simulink model "TV_2021"  (R2017b)
settings: Solver=VariableStepAuto  StartTime=0.0  StopTime=10.0  RelTol=1e-3
undefined symbols (not defined in the file): sigbuilder_block
libraries: simulink x6
(part 4 of 13)

== system TV_2021/If Action Subsystem1/VDC 2018 Complete/Optimization SKF & CKF ==
  RPM_INV1 : Inport
  RPM_INV2 : Inport  Port=2
  Steer_An : Inport  Port=3
  SKF_Initial : Inport  Port=4
  CKF_Initial : Inport  Port=5
  Cte_SKF : Inport  Port=6
  Cte_CKF : Inport  Port=7
  CKF_prev : DataStoreRead  DataStoreName=B
  Constant : Constant  Value=0
  Data Store Memory : DataStoreMemory  ReadBeforeWriteMsg=warning  WriteAfterWriteMsg=warning  WriteAfterReadMsg=warning  ShowAdditionalParam=off
  Data Store Memory1 : DataStoreMemory  DataStoreName=B  ReadBeforeWriteMsg=warning  WriteAfterWriteMsg=warning  WriteAfterReadMsg=warning  ShowAdditionalParam=off
  Data Store Write : DataStoreWrite
  Data Store Write1 : DataStoreWrite  DataStoreName=B
  Derivative : Derivative
  Display : Display
  MATLAB Function : MATLAB Function  TreatAsAtomicUnit=on
  Mux : Mux  Inputs=3
  "SKF_prev " : DataStoreRead
  Saturation : Saturate  UpperLimit=6000  LowerLimit=0
  Scope : Scope
  "Subsystem " : Subsystem
  Switch : Switch  Threshold=900
  SKF_act : Outport
  CKF_act : Outport  Port=2
  wires:
  SKF_Initial/1 -> "Subsystem "/3(SKF_Initial)
  CKF_prev/1 -> "Subsystem "/6("CKF_prev ")
  "Subsystem "/1("SKF_act ") -> SKF_act/1, Data Store Write/1  "SKF"
  Derivative/1 -> Switch/1, Switch/2, Saturation/1, Display/1, "Subsystem "/2(Derivative)  "alpha"
  "SKF_prev "/1 -> "Subsystem "/4(SKF_prev)
  "Subsystem "/2(CKF_act) -> CKF_act/1, Data Store Write1/1  "CKF"
  Cte_CKF/1 -> "Subsystem "/8(Cte_CKF)
  Steer_An/1 -> "Subsystem "/1(Steer_An)
  CKF_Initial/1 -> "Subsystem "/5("CKF_Initial ")
  RPM_INV1/1 -> Mux/1, MATLAB Function/1(RPM_INV1)
  RPM_INV2/1 -> MATLAB Function/2(RPM_INV2)
  Cte_SKF/1 -> "Subsystem "/7(Cte_SKF)
  MATLAB Function/1(RPM) -> Derivative/1  "w (rpm)"
  Mux/1 -> Scope/1
  Saturation/1 -> Mux/2
  Switch/1 -> Mux/3
  Constant/1 -> Switch/3

== system TV_2021/If Action Subsystem1/VDC 2018 Complete/Sensor_DATA ==
  note: [rad/s]
  note: [ºC]
  note: [m/s2]
  note: [m/s2]
  note: [deg]
  note: [N]
  note: [N]
  note: [N]
  note: [N]
  note: [0-1]
  note: [0-1]
  note: [0 or 1]
  note: [0 - Inf]
  note: [rad/s]
  note: [rad/s]
  Steer_Ang : Inport
  "F_Acc " : Inport  Port=2
  R_Acc : Inport  Port=3
  Yaw Rate : Inport  Port=4
  FR_Susp : Inport  Port=5
  FL_Susp : Inport  Port=6
  RR_Susp : Inport  Port=7
  RL_Susp : Inport  Port=8
  Gas Pedal : Inport  Port=9
  Brake Pedal : Inport  Port=10
  Regenerative Enable : Inport  Port=11
  "Power " : Inport  Port=12
  TemperatureIN : Inport  Port=13
  Temperature Motor : Inport  Port=14
  V_eRR : Inport  Port=15
  "V_eRL " : Inport  Port=16
  Steer_ang : Outport
  F_acc : Outport  Port=2
  R_acc : Outport  Port=3
  YawRate : Outport  Port=4
  FR_susp : Outport  Port=5
  FL_susp : Outport  Port=6
  RR_susp : Outport  Port=7
  RL_susp : Outport  Port=8
  Gas_Pedal : Outport  Port=9
  Brake_Pedal : Outport  Port=10
  Reg_Enable : Outport  Port=11
  Power : Outport  Port=12
  TemperatureIGBT : Outport  Port=13
  TemperatureMotor : Outport  Port=14
  "V_eRR " : Outport  Port=15
  V_eRL : Outport  Port=16
  wires:
  RL_Susp/1 -> RL_susp/1
  RR_Susp/1 -> RR_susp/1
  FL_Susp/1 -> FL_susp/1
  FR_Susp/1 -> FR_susp/1
  Steer_Ang/1 -> Steer_ang/1
  R_Acc/1 -> R_acc/1
  "F_Acc "/1 -> F_acc/1
  Gas Pedal/1 -> Gas_Pedal/1
  Brake Pedal/1 -> Brake_Pedal/1
  Regenerative Enable/1 -> Reg_Enable/1
  "Power "/1 -> Power/1
  TemperatureIN/1 -> TemperatureIGBT/1
  "V_eRL "/1 -> V_eRL/1
  V_eRR/1 -> "V_eRR "/1
  Temperature Motor/1 -> TemperatureMotor/1
  Yaw Rate/1 -> YawRate/1

== system TV_2021/If Action Subsystem1/VDC 2018 Complete/Wheel_to_engine ==
  "Fx_FR " : Inport
  "Fx_FL " : Inport  Port=2
  "Fx_RR " : Inport  Port=3
  "Fx_RL " : Inport  Port=4
  Re : Inport  Port=5
  RT : Inport  Port=6
  Add : Sum  Inputs=+-
  Constant : Constant  Value=0
  Constant1 : Constant  Value=0
  Fx_to_engineTqRL : Subsystem
  Fx_to_engineTqRR : Subsystem
  MATLAB Function1 : MATLAB Function  TreatAsAtomicUnit=on
  MATLAB Function2 : MATLAB Function  TreatAsAtomicUnit=on
  Tq_diff : Outport  VectorParamsAs1DForOutWhenUnconnected=on
  Tq_FR : Outport  Port=2
  Tq_FL : Outport  Port=3
  Tq_RR : Outport  Port=4
  Tq_RL : Outport  Port=5
  wires:
  Fx_to_engineTqRR/1(Tq) -> Add/1, Tq_RR/1
  Fx_to_engineTqRL/1(Tq) -> Tq_RL/1, Add/2
  "Fx_FR "/1 -> Tq_FR/1
  "Fx_FL "/1 -> Tq_FL/1
  Re/1 -> Fx_to_engineTqRR/2(Re), Fx_to_engineTqRL/2(Re)
  RT/1 -> Fx_to_engineTqRR/3(RT), Fx_to_engineTqRL/3(RT)
  "Fx_RL "/1 -> MATLAB Function2/2(v)
  "Fx_RR "/1 -> MATLAB Function1/2(v)
  MATLAB Function2/1(value) -> Fx_to_engineTqRL/1(Fx)
  MATLAB Function1/1(value) -> Fx_to_engineTqRR/1(Fx)
  Constant1/1 -> MATLAB Function1/1(cte)
  Constant/1 -> MATLAB Function2/1(cte)
  Add/1 -> Tq_diff/1

== system TV_2021/If Action Subsystem1/VDC 2018 without Longitudinal/Constraints ==
  Tq_FRin : Inport
  Tq_FLin : Inport  Port=2
  Tq_RR_wc : Inport  Port=3
  "Tq_RL_wc " : Inport  Port=4
  "Trans_max_static " : Inport  Port=5
  Trans_max_dynamic : Inport  Port=6
  Power : Inport  Port=7
  Power_limit : Inport  Port=8
  ReductionCte_Power : Inport  Port=9
  ReductionCte_Temperature : Inport  Port=10
  TemperatureIGBT : Inport  Port=11
  TemperatureI_limit_Motor : Inport  Port=12
  TemperatureIMotor : Inport  Port=13
  Temperature_limit_IGBT : Inport  Port=14
  V_eRR : Inport  Port=15
  V_eRL : Inport  Port=16
  Tq_max : Inport  Port=17
  MaxRegTorque : Inport  Port=18
  Bp : Inport  Port=19
  Reg_enable : Inport  Port=20
  Acelerating and braking without Regenerative : Subsystem  TreatAsAtomicUnit=on
  Braking with Regenerative : Subsystem  TreatAsAtomicUnit=on
  Constant : Constant  Value=0
  Constant1 : Constant  Value=0
  If : If  NumInputs=2  IfExpression=u2 == 1 & u1 > 0
  Merge1 : Merge
  Merge2 : Merge
  Tq_FRout : Outport
  "Tq_FLout " : Outport  Port=2
  Tq_RRout : Outport  Port=3
  Tq_RLout : Outport  Port=4
  wires:
  Constant1/1 -> "Tq_FLout "/1
  Constant/1 -> Tq_FRout/1
  Tq_RR_wc/1 -> Braking with Regenerative/2(Tq_RR_wc), Acelerating and braking without Regenerative/16(Tq_RR)
  "Tq_RL_wc "/1 -> Acelerating and braking without Regenerative/17(Tq_RL), Braking with Regenerative/3(Tq_RL_wc)
  Tq_max/1 -> Acelerating and braking without Regenerative/1(Tq_max)
  V_eRL/1 -> Acelerating and braking without Regenerative/3(V_eRL)
  Trans_max_dynamic/1 -> Acelerating and braking without Regenerative/4(Trans_max_dynamic)
  "Trans_max_static "/1 -> Acelerating and braking without Regenerative/5(Trans_max_static)
  Merge2/1 -> Tq_RLout/1
  Merge1/1 -> Tq_RRout/1
  Bp/1 -> If/1
  Reg_enable/1 -> If/2
  V_eRR/1 -> Acelerating and braking without Regenerative/2(V_eRR)
  If/1 -> Braking with Regenerative/Action
  If/2 -> Acelerating and braking without Regenerative/Action
  MaxRegTorque/1 -> Braking with Regenerative/1(MaxRegTorque)
  Tq_FRin/1 -> Acelerating and braking without Regenerative/14(Tq_FR)
  Tq_FLin/1 -> Acelerating and braking without Regenerative/15(Tq_FL)
  ReductionCte_Temperature/1 -> Acelerating and braking without Regenerative/13(ReductionCte_Temperature)
  ReductionCte_Power/1 -> Acelerating and braking without Regenerative/12(ReductionCte_Power)
  TemperatureIGBT/1 -> Acelerating and braking without Regenerative/9(TemperatureIGBT)
  Temperature_limit_IGBT/1 -> Acelerating and braking without Regenerative/8(Temperature_limit_IGBT)
  Power/1 -> Acelerating and braking without Regenerative/7(Power)
  Power_limit/1 -> Acelerating and braking without Regenerative/6(Power_limit)
  Acelerating and braking without Regenerative/2(TQ_RL) -> Merge2/1
  Acelerating and braking without Regenerative/1(TQ_RR) -> Merge1/1
  Braking with Regenerative/1(TQ_RR) -> Merge1/2
  Braking with Regenerative/2(TQ_RL) -> Merge2/2
  TemperatureI_limit_Motor/1 -> Acelerating and braking without Regenerative/10(TemperatureI_limit_Motor)
  TemperatureIMotor/1 -> Acelerating and braking without Regenerative/11(TemperatureMotor)

== system TV_2021/If Action Subsystem1/VDC 2018 without Longitudinal/Driver // CarBehaviours ==
  Tq_FRin : Inport
  Tq_FLin : Inport  Port=2
  Tq_RRin : Inport  Port=3
  "Tq_RLin " : Inport  Port=4
  Bp : Inport  Port=5
  Ap : Inport  Port=6
  Reg_enable : Inport  Port=7
  Ap_Sat_up : Inport  Port=8
  Ap_Sat_down : Inport  Port=9
  Accelerating : Subsystem  TreatAsAtomicUnit=on
  Braking Conditions : If  NumInputs=3  IfExpression=u1>0 & u2==0 & u3==1  ElseIfExpressions=u1>0 & u2==0.02 & u3==0, u1==0.02 & u2==0.02
  Constant : Constant  Value=0
  Constant1 : Constant  Value=0
  Inertia Braking : Subsystem  TreatAsAtomicUnit=on
  Mech_Braking : Subsystem  TreatAsAtomicUnit=on
  Merge : Merge  Inputs=4
  Merge1 : Merge  Inputs=4
  Regenerative+Mech Braking : Subsystem  TreatAsAtomicUnit=on
  Terminator : Terminator
  Terminator1 : Terminator
  Tq_FRout : Outport
  "Tq_FLout " : Outport  Port=2
  Tq_RRout : Outport  Port=3
  Tq_RLout : Outport  Port=4
  out_Throttle : Outport  Port=5
  wires:
  Constant1/1 -> "Tq_FLout "/1
  Constant/1 -> Tq_FRout/1
  Tq_FLin/1 -> Terminator1/1
  Tq_FRin/1 -> Terminator/1
  Merge/1 -> Tq_RRout/1
  Merge1/1 -> Tq_RLout/1
  Bp/1 -> Braking Conditions/1
  Ap/1 -> Accelerating/1(Ap), Braking Conditions/2
  Regenerative+Mech Braking/1("Tq_RR ") -> Merge/1
  Mech_Braking/1("Tq_RR ") -> Merge/2
  Inertia Braking/1("Tq_RR ") -> Merge/3
  Accelerating/1("Tq_RR ") -> Merge/4
  Regenerative+Mech Braking/2(Tq_RL) -> Merge1/1
  Mech_Braking/2(Tq_RL) -> Merge1/2
  Inertia Braking/2(Tq_RL) -> Merge1/3
  Accelerating/2(Tq_RL) -> Merge1/4
  Braking Conditions/1 -> Regenerative+Mech Braking/Action
  Braking Conditions/2 -> Mech_Braking/Action
  Braking Conditions/3 -> Inertia Braking/Action
  Braking Conditions/4 -> Accelerating/Action
  Tq_RRin/1 -> Regenerative+Mech Braking/1(RegTq_RR), Accelerating/4(Tq_RR)
  "Tq_RLin "/1 -> Regenerative+Mech Braking/2(RegTq_RL), Accelerating/5("Tq_RL ")
  Ap_Sat_up/1 -> Accelerating/2("Ap_Sat_up ")
  Ap_Sat_down/1 -> Accelerating/3(Ap_Sat_down)
  Reg_enable/1 -> Braking Conditions/3
  Accelerating/3(Out_Throttle) -> out_Throttle/1

== system TV_2021/If Action Subsystem1/VDC 2018 without Longitudinal/In_Numbers ==
  C-Kamm_Factor : Inport
  Max Regen Torque [Nm] : Inport  Port=2
  Limit Power [kW] : Inport  Port=3
  Limit Temperature IGBT [ºC] : Inport  Port=4
  Limit Temperature Motor [ºC] : Inport  Port=5
  Reduction Power [0-1] : Inport  Port=6
  Reduction Temperature [0-1] : Inport  Port=7
  Steering Saturation (per site) [deg] : Inport  Port=8
  Ap_Sat_Down [-] : Inport  Port=9
  Ap_Sat_Up [-] : Inport  Port=10
  3% difference : Gain  Gain=0.97
  Effective Rolling Radius[inch] : Constant  Value=13
  Engine+Inverter Performance [-] : Constant  Value=0.8
  Maximum Torque per engine [Nm] : Constant  Value=140
  Maximum Transmission Torque Dynamic [Nm] : Constant  Value=140
  Maximum Transmission Torque Static [Nm] : Constant  Value=130
  Transmision Ratio[-] : Constant  Value=4
  inch to m : Gain  Gain=0.0254
  Steer_Sat [deg] : Outport
  Tq_Max [Nm] : Outport  Port=2
  Cornering Kamm_Factor [0-2] : Outport  Port=3
  Transmision_Ratio[-] : Outport  Port=4
  Effective Rolling Radius[m] : Outport  Port=5
  Ap_Sat_down[-] : Outport  Port=6
  Ap_Sat_up[-] : Outport  Port=7
  Engine+Inverter Performance[-] : Outport  Port=8
  Trans_max _static[Nm] : Outport  Port=9
  Trans_max_dynamic [Nm] : Outport  Port=10
  "Power limit [KW] " : Outport  Port=11
  Temperature limit IGBT [ºC] : Outport  Port=12
  Temperature limit Motor [ºC] : Outport  Port=13
  Reduction Power (0-1) : Outport  Port=14
  Reduction Temperature (0-1) : Outport  Port=15
  MaxRegTorque [Nm] : Outport  Port=16
  wires:
  Maximum Torque per engine [Nm]/1 -> Tq_Max [Nm]/1
  Transmision Ratio[-]/1 -> Transmision_Ratio[-]/1
  Effective Rolling Radius[inch]/1 -> inch to m/1
  Maximum Transmission Torque Static [Nm]/1 -> Trans_max _static[Nm]/1
  Maximum Transmission Torque Dynamic [Nm]/1 -> Trans_max_dynamic [Nm]/1
  inch to m/1 -> 3% difference/1
  3% difference/1 -> Effective Rolling Radius[m]/1
  Engine+Inverter Performance [-]/1 -> Engine+Inverter Performance[-]/1
  Max Regen Torque [Nm]/1 -> MaxRegTorque [Nm]/1
  Limit Power [kW]/1 -> "Power limit [KW] "/1
  Limit Temperature IGBT [ºC]/1 -> Temperature limit IGBT [ºC]/1
  Reduction Power [0-1]/1 -> Reduction Power (0-1)/1
  C-Kamm_Factor/1 -> Cornering Kamm_Factor [0-2]/1
  Steering Saturation (per site) [deg]/1 -> Steer_Sat [deg]/1
  Ap_Sat_Up [-]/1 -> Ap_Sat_up[-]/1
  Ap_Sat_Down [-]/1 -> Ap_Sat_down[-]/1
  Reduction Temperature [0-1]/1 -> Reduction Temperature (0-1)/1
  Limit Temperature Motor [ºC]/1 -> Temperature limit Motor [ºC]/1

== system TV_2021/If Action Subsystem1/VDC 2018 without Longitudinal/Kamm Circle Lateral ==
  "N_FR " : Inport
  N_FL : Inport  Port=2
  N_RR : Inport  Port=3
  N_RL : Inport  Port=4
  Fy : Inport  Port=5
  CK_Factor : Inport  Port=6
  Constant : Constant  Value=-1
  Constant1 : Constant  Value=-1
  Kamm_Circle LatD : MATLAB Function  TreatAsAtomicUnit=on
  MATLAB Function1 : MATLAB Function  TreatAsAtomicUnit=on
  MATLAB Function2 : MATLAB Function  TreatAsAtomicUnit=on
  Product : Product
  Product1 : Product
  Fx_FR : Outport
  Fx_FL : Outport  Port=2
  "Fx_RR " : Outport  Port=3
  "Fx_RL " : Outport  Port=4
  wires:
  N_FL/1 -> Fx_FL/1
  "N_FR "/1 -> Fx_FR/1
  N_RL/1 -> Kamm_Circle LatD/2(Fz_L)
  Fy/1 -> Kamm_Circle LatD/3(Fy)
  N_RR/1 -> Kamm_Circle LatD/1(Fz_R)
  Kamm_Circle LatD/1(Fx_R) -> Product/1
  Kamm_Circle LatD/2(Fx_L) -> Product1/1
  CK_Factor/1 -> Product/2, Product1/2
  Product1/1 -> MATLAB Function1/2(v)
  Product/1 -> MATLAB Function2/2(v)
  Constant1/1 -> MATLAB Function2/1(cte)
  MATLAB Function2/1(value) -> "Fx_RR "/1
  Constant/1 -> MATLAB Function1/1(cte)
  MATLAB Function1/1(value) -> "Fx_RL "/1

== system TV_2021/If Action Subsystem1/VDC 2018 without Longitudinal/Lateral Dynamics ==
  F_acc : Inport
  R_acc : Inport  Port=2
  FR_susp : Inport  Port=3
  FL_susp : Inport  Port=4
  RR_susp : Inport  Port=5
  RL_susp : Inport  Port=6
  Gas_pedal : Inport  Port=7
  Brake_pedal : Inport  Port=8
  Constant1 : Constant  Value=0
  Constant2 : Constant  Value=0
  Demux : Demux  Outputs=3
  Demux1 : Demux  Outputs=3
  Fy per wheel : Gain  Gain=1/2
  Gravity : Gain  Gain=1/9.81
  Gravity1 : Gain  Gain=1/9.81
  Product : Product
  Sum : Sum  Inputs=++++
  Sum1 : Sum
  Sum2 : Sum  Inputs=+-
  Terminator{1..6} (6 alike) : Terminator
  N_FR : Outport
  "N_FL " : Outport  Port=2
  "N_RR " : Outport  Port=3
  N_RL : Outport  Port=4
  Fy_R : Outport  Port=5
  Mass [kg] (0,inf) : Outport  Port=6
  Handling [-] (-inf,inf) : Outport  Port=7
  wires:
  Constant2/1 -> "N_FL "/1
  Constant1/1 -> N_FR/1
  FL_susp/1 -> Sum/2
  F_acc/1 -> Demux1/1
  RR_susp/1 -> Sum/3, Sum1/1, "N_RR "/1
  RL_susp/1 -> Sum/4, Sum1/2, N_RL/1
  Gas_pedal/1 -> Terminator4/1
  Brake_pedal/1 -> Terminator5/1
  R_acc/1 -> Demux/1
  Demux/2 -> Sum2/2, Product/1
  Demux/1 -> Terminator6/1
  Demux/3 -> Terminator3/1
  Product/1 -> Fy per wheel/1  "Fy per axe"
  Fy per wheel/1 -> Fy_R/1
  Gravity1/1 -> Product/2
  Sum/1 -> Gravity/1
  FR_susp/1 -> Sum/1
  Sum1/1 -> Gravity1/1
  Gravity/1 -> Mass [kg] (0,inf)/1  "Mass [kg]"
  Demux1/1 -> Terminator1/1
  Demux1/3 -> Terminator2/1
  Demux1/2 -> Sum2/1
  Sum2/1 -> Handling [-] (-inf,inf)/1

== system TV_2021/If Action Subsystem1/VDC 2018 without Longitudinal/Optimization SKF & CKF ==
  RPM_INV1 : Inport
  RPM_INV2 : Inport  Port=2
  CKF_Initial : Inport  Port=3
  Cte_CKF : Inport  Port=4
  CKF_prev : DataStoreRead  DataStoreName=B
  Data Store Memory1 : DataStoreMemory  DataStoreName=B  ReadBeforeWriteMsg=warning  WriteAfterWriteMsg=warning  WriteAfterReadMsg=warning  ShowAdditionalParam=off
  Data Store Write1 : DataStoreWrite  DataStoreName=B
  Derivative : Derivative
  MATLAB Function : MATLAB Function  TreatAsAtomicUnit=on
  "Subsystem " : Subsystem
  CKF_act : Outport
  wires:
  CKF_prev/1 -> "Subsystem "/3("CKF_prev ")
  Derivative/1 -> "Subsystem "/1(Derivative)  "alpha"
  MATLAB Function/1(RPM) -> Derivative/1  "w (rpm)"
  "Subsystem "/1(CKF_act) -> Data Store Write1/1, CKF_act/1  "CKF"
  Cte_CKF/1 -> "Subsystem "/4(Cte_CKF)
  CKF_Initial/1 -> "Subsystem "/2("CKF_Initial ")
  RPM_INV1/1 -> MATLAB Function/1(RPM_INV1)
  RPM_INV2/1 -> MATLAB Function/2(RPM_INV2)

== system TV_2021/If Action Subsystem1/VDC 2018 without Longitudinal/Sensor_DATA ==
  note: [ºC]
  note: [m/s2]
  note: [m/s2]
  note: [deg]
  note: [N]
  note: [N]
  note: [N]
  note: [N]
  note: [0-1]
  note: [0-1]
  note: [0 or 1]
  note: [0 - Inf]
  note: [rad/s]
  note: [rad/s]
  Steer_Ang : Inport
  "F_Acc " : Inport  Port=2
  R_Acc : Inport  Port=3
  FR_Susp : Inport  Port=4
  FL_Susp : Inport  Port=5
  RR_Susp : Inport  Port=6
  RL_Susp : Inport  Port=7
  Gas Pedal : Inport  Port=8
  Brake Pedal : Inport  Port=9
  Regenerative Enable : Inport  Port=10
  "Power " : Inport  Port=11
  TemperatureIGBT : Inport  Port=12
  TemperatureMotor : Inport  Port=13
  V_eRR : Inport  Port=14
  "V_eRL " : Inport  Port=15
  Steer_ang : Outport
  F_acc : Outport  Port=2
  R_acc : Outport  Port=3
  FR_susp : Outport  Port=4
  FL_susp : Outport  Port=5
  RR_susp : Outport  Port=6
  RL_susp : Outport  Port=7
  Gas_Pedal : Outport  Port=8
  Brake_Pedal : Outport  Port=9
  Reg_Enable : Outport  Port=10
  Power : Outport  Port=11
  Temperature IGBT : Outport  Port=12
  Temperature Motor : Outport  Port=13
  "V_eRR " : Outport  Port=14
  V_eRL : Outport  Port=15
  wires:
  RL_Susp/1 -> RL_susp/1
  RR_Susp/1 -> RR_susp/1
  FL_Susp/1 -> FL_susp/1
  FR_Susp/1 -> FR_susp/1
  Steer_Ang/1 -> Steer_ang/1
  R_Acc/1 -> R_acc/1
  "F_Acc "/1 -> F_acc/1
  Gas Pedal/1 -> Gas_Pedal/1
  Brake Pedal/1 -> Brake_Pedal/1
  Regenerative Enable/1 -> Reg_Enable/1
  "Power "/1 -> Power/1
  TemperatureIGBT/1 -> Temperature IGBT/1
  "V_eRL "/1 -> V_eRL/1
  V_eRR/1 -> "V_eRR "/1
  TemperatureMotor/1 -> Temperature Motor/1

== system TV_2021/If Action Subsystem1/VDC 2018 without Longitudinal/Wheel_to_engine ==
  "Fx_FR " : Inport
  "Fx_FL " : Inport  Port=2
  "Fx_RR " : Inport  Port=3
  "Fx_RL " : Inport  Port=4
  Re : Inport  Port=5
  RT : Inport  Port=6
  Constant : Constant  Value=0
  Constant1 : Constant  Value=0
  Fx_to_engineTqRL : Subsystem
  Fx_to_engineTqRR : Subsystem
  MATLAB Function1 : MATLAB Function  TreatAsAtomicUnit=on
  MATLAB Function2 : MATLAB Function  TreatAsAtomicUnit=on
  Tq_FR : Outport
  Tq_FL : Outport  Port=2
  Tq_RR : Outport  Port=3
  Tq_RL : Outport  Port=4
  wires:
  Fx_to_engineTqRR/1(Tq) -> Tq_RR/1
  Fx_to_engineTqRL/1(Tq) -> Tq_RL/1
  "Fx_FR "/1 -> Tq_FR/1
  "Fx_FL "/1 -> Tq_FL/1
  Re/1 -> Fx_to_engineTqRR/2(Re), Fx_to_engineTqRL/2(Re)
  RT/1 -> Fx_to_engineTqRR/3(RT), Fx_to_engineTqRL/3(RT)
  "Fx_RR "/1 -> MATLAB Function2/2(v)
  "Fx_RL "/1 -> MATLAB Function1/2(v)
  MATLAB Function2/1(value) -> Fx_to_engineTqRR/1(Fx)
  Constant/1 -> MATLAB Function2/1(cte)
  Constant1/1 -> MATLAB Function1/1(cte)
  MATLAB Function1/1(value) -> Fx_to_engineTqRL/1(Fx)

== system TV_2021/Vehicle Dynamics Control 1/Rigid Axle/Accelerating ==
  Ap : Inport
  "Ap_Sat_up " : Inport  Port=2
  Ap_Sat_down : Inport  Port=3
  Tq_RR : Inport  Port=4
  "Tq_RL " : Inport  Port=5
  "Accelerator behaviour " : MATLAB Function  TreatAsAtomicUnit=on
  Product : Product
  Product1 : Product
  "Tq_RR " : Outport
  Tq_RL : Outport  Port=2
  wires:
  Product1/1 -> "Tq_RR "/1
  "Tq_RL "/1 -> Product/2
  Tq_RR/1 -> Product1/2
  Ap/1 -> "Accelerator behaviour "/1(Ap)
  "Ap_Sat_up "/1 -> "Accelerator behaviour "/2(Ap_Sat_up)
  "Accelerator behaviour "/1(throttle) -> Product1/1, Product/1
  Product/1 -> Tq_RL/1
  Ap_Sat_down/1 -> "Accelerator behaviour "/3(Ap_Sat_down)

== system TV_2021/Vehicle Dynamics Control 1/Steering TV 2017 with TC/Accelerating ==
  Ap : Inport
  "Ap_Sat_up " : Inport  Port=2
  Ap_Sat_down : Inport  Port=3
  Tq_RR : Inport  Port=4
  "Tq_RL " : Inport  Port=5
  "Accelerator behaviour " : MATLAB Function  TreatAsAtomicUnit=on
  Product : Product
  Product1 : Product
  "Tq_RR " : Outport
  Tq_RL : Outport  Port=2
  wires:
  Product1/1 -> "Tq_RR "/1
  "Tq_RL "/1 -> Product/2
  Tq_RR/1 -> Product1/2
  Ap/1 -> "Accelerator behaviour "/1(Ap)
  "Ap_Sat_up "/1 -> "Accelerator behaviour "/2(Ap_Sat_up)
  "Accelerator behaviour "/1(throttle) -> Product1/1, Product/1
  Product/1 -> Tq_RL/1
  Ap_Sat_down/1 -> "Accelerator behaviour "/3(Ap_Sat_down)

== system TV_2021/Vehicle Dynamics Control 1/Steering TV 2017 with TC/Constraints ==
  note: Considero de la misma gravedad,
      | la limitacion por potencia que por temperatura
  Power : Inport
  Temperature_limit_IGBT : Inport  Port=2
  Temperature_IGBT : Inport  Port=3
  Temperature_limit_Motor : Inport  Port=4
  Temperature_Motor : Inport  Port=5
  Temp_Celdas : Inport  Port=6
  Lim_Temp_Celdas : Inport  Port=7
  Tq_RR : Inport  Port=8
  Tq_RL : Inport  Port=9
  ReductionCte_Temperature : Inport  Port=10
  ReductionCte_Power : Inport  Port=11
  Voltage : Inport  Port=12
  Corriente : Inport  Port=13
  Constant : Constant  Value=80
  "Control de Potencia " : Subsystem  TreatAsAtomicUnit=on
  Control de Temperatura : Subsystem  TreatAsAtomicUnit=on
  If : If  NumInputs=8  IfExpression=u4 >= u3 | u6 >= u5 | u7>=u8  ElseIfExpressions=u2 >= u1
  Initial Limitation : Constant  Value=0.3
  Merge : Merge  Inputs=3
  Merge1 : Merge  Inputs=3
  Máxima corriente : Constant  Value=140
  Máxima corriente Regenerativa : Constant  Value=0
  Product : Product
  Terminator : Terminator
  Terminator1 : Terminator
  Terminator2 : Terminator
  current_limitation1 : Subsystem
  else : Subsystem  TreatAsAtomicUnit=on
  TQ_RR : Outport
  TQ_RL : Outport  Port=2
  wires:
  Constant/1 -> If/1
  Product/1 -> Terminator2/1  "Powerlimite"
  Initial Limitation/1 -> current_limitation1/3(initial_limitation)
  Corriente/1 -> current_limitation1/2(actual_current)
  [Temp_Celda] -> current_limitation1/1(max_cell_temp)
  Máxima corriente/1 -> current_limitation1/4(max_discharge_current)
  Máxima corriente Regenerativa/1 -> current_limitation1/5(max_regen_current)
  Voltage/1 -> Product/1
  current_limitation1/1(max_discharge (-)) -> Product/2
  current_limitation1/2(max_regen (+)) -> Terminator1/1
  current_limitation1/3(fans_control) -> Terminator/1
  Lim_Temp_Celdas/1 -> If/8
  Temp_Celdas/1 -> If/7, [Temp_Celda]
  Temperature_IGBT/1 -> If/4
  Merge1/1 -> TQ_RL/1
  Merge/1 -> TQ_RR/1
  Temperature_Motor/1 -> If/6
  Temperature_limit_Motor/1 -> If/5
  Control de Temperatura/2(Tq_RL_out) -> Merge1/2
  else/1(Tq_RR_out) -> Merge/3
  Control de Temperatura/1(Tq_RR_out) -> Merge/2
  If/3 -> else/Action
  If/2 -> "Control de Potencia "/Action
  Tq_RL/1 -> else/2(Tq_RL), "Control de Potencia "/2(Tq_RL), Control de Temperatura/2(Tq_RL)
  Tq_RR/1 -> "Control de Potencia "/1(Tq_RR), Control de Temperatura/1(Tq_RR), else/1(Tq_RR)
  If/1 -> Control de Temperatura/Action
  else/2(Tq_RL_out) -> Merge1/3
  "Control de Potencia "/2(Tq_RL_out) -> Merge1/1
  "Control de Potencia "/1(Tq_RR_out) -> Merge/1
  Power/1 -> If/2
  ReductionCte_Temperature/1 -> Control de Temperatura/3(ReductionCte)
  Temperature_limit_IGBT/1 -> If/3
  ReductionCte_Power/1 -> "Control de Potencia "/3(ReductionCte)

== system TV_2021/Vehicle Dynamics Control 1/Steering TV 2017 with TC/Lateral Dynamics ==
  CKF : Inport
  Tq_RR : Inport  Port=2
  Tq_RL : Inport  Port=3
  Action Port : ActionPort
  Product : Product
  Product1 : Product
  Tq_RR_with_CKF : Outport
  Tq_RL_with_CKF : Outport  Port=2
  wires:
  Product/1 -> Tq_RR_with_CKF/1
  CKF/1 -> Product1/2, Product/2
  Tq_RL/1 -> Product1/1
  Tq_RR/1 -> Product/1
  Product1/1 -> Tq_RL_with_CKF/1

== system TV_2021/Vehicle Dynamics Control 1/Steering TV 2017 with TC/Longitudinal Dynamics ==
  SKF : Inport
  Tq_RR : Inport  Port=2
  Tq_RL : Inport  Port=3
  Action Port : ActionPort
  Product : Product
  Product1 : Product
  Tq_RR_with_SKF : Outport
  Tq_RL_with_SKF : Outport  Port=2
  wires:
  Product1/1 -> Tq_RL_with_SKF/1
  Product/1 -> Tq_RR_with_SKF/1
  SKF/1 -> Product1/2, Product/2
  Tq_RL/1 -> Product1/1
  Tq_RR/1 -> Product/1

== system TV_2021/Vehicle Dynamics Control 1/Steering TV 2017 with TC/Optimization SKF & CKF ==
  RPM_INV1 : Inport
  RPM_INV2 : Inport  Port=2
  Steer_An : Inport  Port=3
  SKF_Initial : Inport  Port=4
  CKF_Initial : Inport  Port=5
  Cte_SKF : Inport  Port=6
  Cte_CKF : Inport  Port=7
  CKF_prev : DataStoreRead  DataStoreName=B
  Constant : Constant  Value=0
  Data Store Memory : DataStoreMemory  ReadBeforeWriteMsg=warning  WriteAfterWriteMsg=warning  WriteAfterReadMsg=warning  ShowAdditionalParam=off
  Data Store Memory1 : DataStoreMemory  DataStoreName=B  ReadBeforeWriteMsg=warning  WriteAfterWriteMsg=warning  WriteAfterReadMsg=warning  ShowAdditionalParam=off
  Data Store Write : DataStoreWrite
  Data Store Write1 : DataStoreWrite  DataStoreName=B
  Derivative : Derivative
  Display : Display
  MATLAB Function : MATLAB Function  TreatAsAtomicUnit=on
  Mux : Mux  Inputs=3
  "SKF_prev " : DataStoreRead
  Saturation : Saturate  UpperLimit=6000  LowerLimit=0
  Scope{,1,3..5} (5 alike) : Scope
  Scope2 : Scope  NumInputPorts=2
  Scope7 : Scope  NumInputPorts=3
  Signal Generator : SignalGenerator  WaveForm=square  Units=rad/sec
  Sine Wave : Sin  SampleTime=0
  "Subsystem " : Subsystem
  Switch : Switch  Threshold=900
  SKF_act : Outport
  CKF_act : Outport  Port=2
  wires:
  RPM_INV2/1 -> Scope2/1, MATLAB Function/2(RPM_INV2), Scope3/1
  CKF_prev/1 -> "Subsystem "/6("CKF_prev ")
  Sine Wave/1 -> Scope5/1
  Signal Generator/1 -> Scope4/1
  "SKF_prev "/1 -> "Subsystem "/4(SKF_prev)
  RPM_INV1/1 -> Mux/1, MATLAB Function/1(RPM_INV1)
  Constant/1 -> Switch/3
  Switch/1 -> Mux/3
  Saturation/1 -> Mux/2
  Mux/1 -> Scope/1
  MATLAB Function/1(RPM) -> Derivative/1, Scope1/1, Scope7/3  "w (rad/s)"
  Cte_SKF/1 -> "Subsystem "/7(Cte_SKF)
  CKF_Initial/1 -> "Subsystem "/5("CKF_Initial ")
  Steer_An/1 -> "Subsystem "/1(Steer_An)
  Cte_CKF/1 -> "Subsystem "/8(Cte_CKF)
  "Subsystem "/2(CKF_act) -> Data Store Write1/1, Scope7/1, CKF_act/1  "CKF"
  Derivative/1 -> Saturation/1, Switch/2, Switch/1, "Subsystem "/2(Derivative), Display/1, Scope7/2, Scope2/2  "alpha"
  "Subsystem "/1("SKF_act ") -> Data Store Write/1, SKF_act/1  "SKF"
  SKF_Initial/1 -> "Subsystem "/3(SKF_Initial)

== system TV_2021/Vehicle Dynamics Control 1/VDC 2018 Complete/Constraints ==
  Tq_FRin : Inport
  Tq_FLin : Inport  Port=2
  Tq_RR_wc : Inport  Port=3
  "Tq_RL_wc " : Inport  Port=4
  "Trans_max_static " : Inport  Port=5
  Trans_max_dynamic : Inport  Port=6
  Power : Inport  Port=7
  Power_limit : Inport  Port=8
  ReductionCte_Power : Inport  Port=9
  ReductionCte_Temperature : Inport  Port=10
  TemperatureIGBT : Inport  Port=11
  TemperatureI_limit_Motor : Inport  Port=12
  TemperatureIMotor : Inport  Port=13
  Temperature_limit_IGBT : Inport  Port=14
  V_eRR : Inport  Port=15
  V_eRL : Inport  Port=16
  Tq_max : Inport  Port=17
  MaxRegTorque : Inport  Port=18
  Bp : Inport  Port=19
  Reg_enable : Inport  Port=20
  Tq_diff : Inport  Port=21
  Tq_diff_max : Inport  Port=22
  Temp_celdas : Inport  Port=23
  Limit_Temp_celdas : Inport  Port=24
  Acelerating and braking without Regenerative : Subsystem  TreatAsAtomicUnit=on
  Braking with Regenerative : Subsystem  TreatAsAtomicUnit=on
  Constant : Constant  Value=0
  Constant1 : Constant  Value=0
  If : If  NumInputs=2  IfExpression=u2 == 1 & u1 > 0
  Merge1 : Merge
  Merge2 : Merge
  Tq_FRout : Outport
  "Tq_FLout " : Outport  Port=2
  Tq_RRout : Outport  Port=3
  Tq_RLout : Outport  Port=4
  Flag_Temperature : Outport  Port=5
  Flag_Power : Outport  Port=6
  wires:
  Limit_Temp_celdas/1 -> Acelerating and braking without Regenerative/21(Limit_Temp_celdas)
  Temp_celdas/1 -> Acelerating and braking without Regenerative/20(Temp_celdas)
  Tq_diff_max/1 -> Acelerating and braking without Regenerative/19(Tq_diff_max)
  Tq_diff/1 -> Acelerating and braking without Regenerative/18(Tq_diff)
  Acelerating and braking without Regenerative/3(Flag_Temperature) -> Flag_Temperature/1
  Acelerating and braking without Regenerative/4(Flag_Power) -> Flag_Power/1
  TemperatureIMotor/1 -> Acelerating and braking without Regenerative/11(TemperatureMotor)
  TemperatureI_limit_Motor/1 -> Acelerating and braking without Regenerative/10(TemperatureI_limit_Motor)
  Braking with Regenerative/2(TQ_RL) -> Merge2/2
  Braking with Regenerative/1(TQ_RR) -> Merge1/2
  Acelerating and braking without Regenerative/1(TQ_RR) -> Merge1/1
  Acelerating and braking without Regenerative/2(TQ_RL) -> Merge2/1
  Power_limit/1 -> Acelerating and braking without Regenerative/6(Power_limit)
  Power/1 -> Acelerating and braking without Regenerative/7(Power)
  Temperature_limit_IGBT/1 -> Acelerating and braking without Regenerative/8(Temperature_limit_IGBT)
  TemperatureIGBT/1 -> Acelerating and braking without Regenerative/9(TemperatureIGBT)
  ReductionCte_Power/1 -> Acelerating and braking without Regenerative/12(ReductionCte_Power)
  ReductionCte_Temperature/1 -> Acelerating and braking without Regenerative/13(ReductionCte_Temperature)
  Tq_FLin/1 -> Acelerating and braking without Regenerative/15(Tq_FL)
  Tq_FRin/1 -> Acelerating and braking without Regenerative/14(Tq_FR)
  MaxRegTorque/1 -> Braking with Regenerative/1(MaxRegTorque)
  If/2 -> Acelerating and braking without Regenerative/Action
  If/1 -> Braking with Regenerative/Action
  V_eRR/1 -> Acelerating and braking without Regenerative/2(V_eRR)
  Reg_enable/1 -> If/2
  Bp/1 -> If/1
  Merge1/1 -> Tq_RRout/1
  Merge2/1 -> Tq_RLout/1
  "Trans_max_static "/1 -> Acelerating and braking without Regenerative/5(Trans_max_static)
  Trans_max_dynamic/1 -> Acelerating and braking without Regenerative/4(Trans_max_dynamic)
  V_eRL/1 -> Acelerating and braking without Regenerative/3(V_eRL)
  Tq_max/1 -> Acelerating and braking without Regenerative/1(Tq_max)
  "Tq_RL_wc "/1 -> Acelerating and braking without Regenerative/17(Tq_RL), Braking with Regenerative/3(Tq_RL_wc)
  Tq_RR_wc/1 -> Acelerating and braking without Regenerative/16(Tq_RR), Braking with Regenerative/2(Tq_RR_wc)
  Constant/1 -> Tq_FRout/1
  Constant1/1 -> "Tq_FLout "/1

== system TV_2021/Vehicle Dynamics Control 1/VDC 2018 Complete/Driver // CarBehaviours ==
  Tq_FRin : Inport
  Tq_FLin : Inport  Port=2
  Tq_RRin : Inport  Port=3
  "Tq_RLin " : Inport  Port=4
  Bp : Inport  Port=5
  Ap : Inport  Port=6
  Reg_enable : Inport  Port=7
  Ap_Sat_up : Inport  Port=8
  Ap_Sat_down : Inport  Port=9
  Accelerating : Subsystem  TreatAsAtomicUnit=on
  "Accelerator behaviour " : MATLAB Function  TreatAsAtomicUnit=on
  Braking Conditions : If  NumInputs=3  IfExpression=u1>0 & u2<0.1 & u3==1  ElseIfExpressions=u1>0 & u2<0.1 & u3==0, u1<0.1 & u2<0.1
  Constant : Constant  Value=0
  Constant1 : Constant  Value=0
  Inertia Braking : Subsystem  TreatAsAtomicUnit=on
  Mech_Braking : Subsystem  TreatAsAtomicUnit=on
  Merge : Merge  Inputs=4
  Merge1 : Merge  Inputs=4
  Regenerative+Mech Braking : Subsystem  TreatAsAtomicUnit=on
  Terminator : Terminator
  Terminator1 : Terminator
  Tq_FRout : Outport
  "Tq_FLout " : Outport  Port=2
  Tq_RRout : Outport  Port=3
  Tq_RLout : Outport  Port=4
  out_Throttle : Outport  Port=5
  wires:
  Ap_Sat_down/1 -> "Accelerator behaviour "/3(Ap_Sat_down)
  Ap_Sat_up/1 -> "Accelerator behaviour "/2(Ap_Sat_up)
  Ap/1 -> "Accelerator behaviour "/1(Ap)
  "Accelerator behaviour "/1(throttle) -> Braking Conditions/2, Accelerating/1(Throttle)
  Accelerating/3(Out_Throttle) -> out_Throttle/1
  Reg_enable/1 -> Braking Conditions/3
  "Tq_RLin "/1 -> Regenerative+Mech Braking/2(RegTq_RL), Accelerating/3("Tq_RL ")
  Tq_RRin/1 -> Regenerative+Mech Braking/1(RegTq_RR), Accelerating/2(Tq_RR)
  Braking Conditions/4 -> Accelerating/Action
  Braking Conditions/3 -> Inertia Braking/Action
  Braking Conditions/2 -> Mech_Braking/Action
  Braking Conditions/1 -> Regenerative+Mech Braking/Action
  Accelerating/2(Tq_RL) -> Merge1/4
  Inertia Braking/2(Tq_RL) -> Merge1/3
  Mech_Braking/2(Tq_RL) -> Merge1/2
  Regenerative+Mech Braking/2(Tq_RL) -> Merge1/1
  Accelerating/1("Tq_RR ") -> Merge/4
  Inertia Braking/1("Tq_RR ") -> Merge/3
  Mech_Braking/1("Tq_RR ") -> Merge/2
  Regenerative+Mech Braking/1("Tq_RR ") -> Merge/1
  Bp/1 -> Braking Conditions/1
  Merge1/1 -> Tq_RLout/1
  Merge/1 -> Tq_RRout/1
  Tq_FRin/1 -> Terminator/1
  Tq_FLin/1 -> Terminator1/1
  Constant/1 -> Tq_FRout/1
  Constant1/1 -> "Tq_FLout "/1

== system TV_2021/Vehicle Dynamics Control 1/VDC 2018 Complete/Flags ==
  Flag_CarBehavior : Inport
  Flag_WheelSpin_RR : Inport  Port=2
  Flag_WheelSpin_RL : Inport  Port=3
  Flag_Temperature : Inport  Port=4
  Flag_Power : Inport  Port=5
  Mux : Mux  Inputs=5
  Flags : Outport
  wires:
  Flag_Power/1 -> Mux/5
  Flag_Temperature/1 -> Mux/4
  Flag_WheelSpin_RL/1 -> Mux/3
  Flag_WheelSpin_RR/1 -> Mux/2
  Flag_CarBehavior/1 -> Mux/1
  Mux/1 -> Flags/1

== system TV_2021/Vehicle Dynamics Control 1/VDC 2018 Complete/In_Numbers ==
  S-Kamm_Factor : Inport
  C-Kamm_Factor : Inport  Port=2
  Max Regen Torque [Nm] : Inport  Port=3
  Limit Power [kW] : Inport  Port=4
  Limit TemperatureIGBT [ºC] : Inport  Port=5
  Limit Temperature Motor [ºC] : Inport  Port=6
  Reduction_P [0-1] : Inport  Port=7
  Reduction_T [0-1] : Inport  Port=8
  Steering Saturation (per site) [deg] : Inport  Port=9
  Ap_Sat_Up [-] : Inport  Port=10
  Ap_Sat_Down [-] : Inport  Port=11
  3% difference : Gain  Gain=0.97
  360/(2*pi) : Gain  Gain=360/(2*pi)
  Constant1 : Constant  Value=0.025
  Cornering_Stiffness [N/º] : Constant  Value=750
  Effective Rolling Radius[inch] : Constant  Value=13
  Engine+Inverter Performance [-] : Constant  Value=0.8
  Maximum Torque per engine [Nm] : Constant  Value=140
  Maximum Transmission Torque Dynamic [Nm] : Constant  Value=140
  Maximum Transmission Torque Static [Nm] : Constant  Value=130
  "Rear_Trackwidth [m] " : Constant  Value=1.15
  Steering_Ratio [-] : Constant  Value=3.27
  Terminator{,1..4} (5 alike) : Terminator
  Tq_diff_Max : Constant  Value=100
  Transmision Ratio[-] : Constant  Value=4
  Wheelbase [m] : Constant  Value=1.535
  Yaw_Inertia [kg/m^3] : Constant  Value=43.21  VectorParams1D=off  SampleTime=-1
  inch to m : Gain  Gain=0.0254
  Steer_Sat [deg] : Outport
  Tq_Max [Nm] : Outport  Port=2
  Straight Kamm_Factor [0-2] : Outport  Port=3
  Cornering Kamm_Factor [0-2] : Outport  Port=4
  Transmision_Ratio[-] : Outport  Port=5
  Effective Rolling Radius[m] : Outport  Port=6
  Ap_Sat_down[-] : Outport  Port=7
  Ap_Sat_up[-] : Outport  Port=8
  Engine+Inverter Performance[-] : Outport  Port=9
  Trans_max _static[Nm] : Outport  Port=10
  Trans_max_dynamic [Nm] : Outport  Port=11
  "Power limit [KW] " : Outport  Port=12
  Temperature limit IGBT [ºC] : Outport  Port=13
  Temperature limit Motor [ºC] : Outport  Port=14
  ReductionCte_Power (0-1) : Outport  Port=15
  ReductionCte_Temperature (0-1) : Outport  Port=16
  MaxRegTorque [Nm] : Outport  Port=17
  Tq_diff_Max [Nm] : Outport  Port=18  VectorParamsAs1DForOutWhenUnconnected=on
  Yaw_error_correction_time [s] : Outport  Port=19  VectorParamsAs1DForOutWhenUnconnected=on
  wires:
  Constant1/1 -> Yaw_error_correction_time [s]/1
  Tq_diff_Max/1 -> Tq_diff_Max [Nm]/1
  Yaw_Inertia [kg/m^3]/1 -> Terminator4/1
  360/(2*pi)/1 -> Terminator2/1
  Wheelbase [m]/1 -> Terminator3/1
  Cornering_Stiffness [N/º]/1 -> 360/(2*pi)/1
  "Rear_Trackwidth [m] "/1 -> Terminator1/1
  Steering_Ratio [-]/1 -> Terminator/1
  Limit Temperature Motor [ºC]/1 -> Temperature limit Motor [ºC]/1
  Reduction_T [0-1]/1 -> ReductionCte_Temperature (0-1)/1
  Ap_Sat_Down [-]/1 -> Ap_Sat_down[-]/1
  Ap_Sat_Up [-]/1 -> Ap_Sat_up[-]/1
  Steering Saturation (per site) [deg]/1 -> Steer_Sat [deg]/1
  C-Kamm_Factor/1 -> Cornering Kamm_Factor [0-2]/1
  Reduction_P [0-1]/1 -> ReductionCte_Power (0-1)/1
  Limit TemperatureIGBT [ºC]/1 -> Temperature limit IGBT [ºC]/1
  Limit Power [kW]/1 -> "Power limit [KW] "/1
  Max Regen Torque [Nm]/1 -> MaxRegTorque [Nm]/1
  S-Kamm_Factor/1 -> Straight Kamm_Factor [0-2]/1
  Engine+Inverter Performance [-]/1 -> Engine+Inverter Performance[-]/1
  3% difference/1 -> Effective Rolling Radius[m]/1
  inch to m/1 -> 3% difference/1
  Maximum Transmission Torque Dynamic [Nm]/1 -> Trans_max_dynamic [Nm]/1
  Maximum Transmission Torque Static [Nm]/1 -> Trans_max _static[Nm]/1
  Effective Rolling Radius[inch]/1 -> inch to m/1
  Transmision Ratio[-]/1 -> Transmision_Ratio[-]/1
  Maximum Torque per engine [Nm]/1 -> Tq_Max [Nm]/1

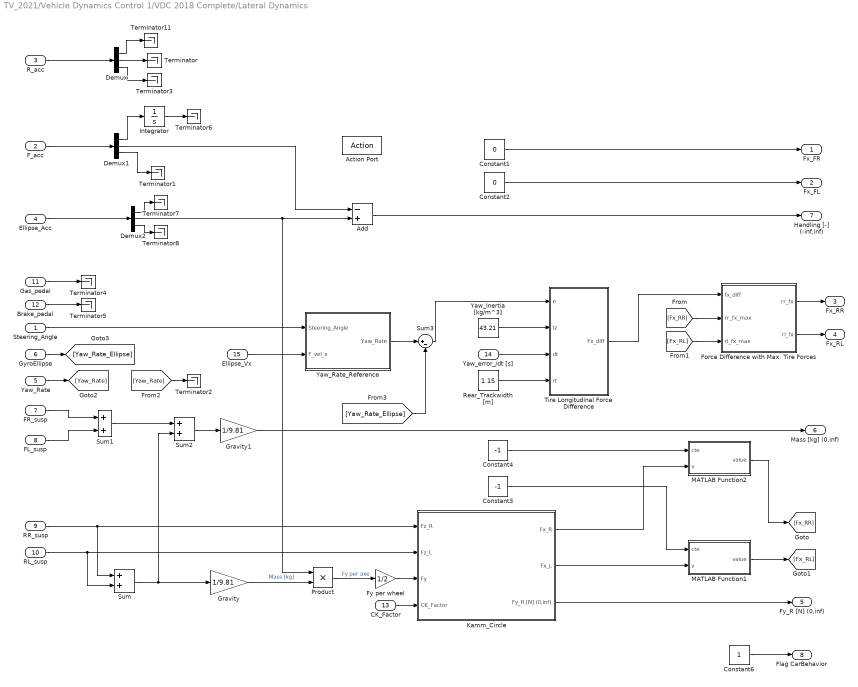
== system TV_2021/Vehicle Dynamics Control 1/VDC 2018 Complete/Lateral Dynamics ==
  Steering_Angle : Inport
  F_acc : Inport  Port=2
  R_acc : Inport  Port=3
  Ellipse_Acc : Inport  Port=4
  Yaw_Rate : Inport  Port=5
  GyroEllipse : Inport  Port=6
  FR_susp : Inport  Port=7
  FL_susp : Inport  Port=8
  RR_susp : Inport  Port=9
  RL_susp : Inport  Port=10
  Gas_pedal : Inport  Port=11
  Brake_pedal : Inport  Port=12
  CK_Factor : Inport  Port=13
  Yaw_error_/dt [s] : Inport  Port=14
  Ellipse_Vx : Inport  Port=15
  Action Port : ActionPort
  Add : Sum  Inputs=-+
  Constant1 : Constant  Value=0
  Constant2 : Constant  Value=0
  Constant3 : Constant  Value=-1
  Constant4 : Constant  Value=-1
  Constant6 : Constant
  Demux : Demux  Outputs=3
  Demux1 : Demux  Outputs=3
  Demux2 : Demux  Outputs=3
  Force Difference with Max. Tire Forces : MATLAB Function  TreatAsAtomicUnit=on
  Fy per wheel : Gain  Gain=1/2
  Gravity : Gain  Gain=1/9.81
  Gravity1 : Gain  Gain=1/9.81
  Integrator : Integrator
  Kamm_Circle : Subsystem
  MATLAB Function1 : MATLAB Function  TreatAsAtomicUnit=on
  MATLAB Function2 : MATLAB Function  TreatAsAtomicUnit=on
  Product : Product
  "Rear_Trackwidth [m] " : Constant  Value=1.15
  Sum : Sum
  Sum1 : Sum
  Sum2 : Sum
  Sum3 : Sum  Inputs=|+-
  Terminator{,1..8,11} (10 alike) : Terminator
  Tire Longitudinal Force Difference : Subsystem
  Yaw_Inertia [kg/m^3] : Constant  Value=43.21  VectorParams1D=off  SampleTime=-1
  Yaw_Rate_Reference : Subsystem
  Fx_FR : Outport
  Fx_FL : Outport  Port=2
  "Fx_RR " : Outport  Port=3
  "Fx_RL " : Outport  Port=4
  Fy_R [N] (0,inf) : Outport  Port=5
  " Mass [kg] (0,inf)" : Outport  Port=6
  Handling [-] (-inf,inf) : Outport  Port=7
  Flag CarBehavior : Outport  Port=8
  wires:
  Demux2/1 -> Terminator7/1
  Demux2/3 -> Terminator8/1
  Demux2/2 -> Add/2, Product/1
  Ellipse_Vx/1 -> Yaw_Rate_Reference/2(F_vel_x)
  Integrator/1 -> Terminator6/1
  [Yaw_Rate] -> Terminator2/1
  GyroEllipse/1 -> [Yaw_Rate_Ellipse]
  Demux/2 -> Terminator/1
  Ellipse_Acc/1 -> Demux2/1
  Gas_pedal/1 -> Terminator4/1
  Brake_pedal/1 -> Terminator5/1
  R_acc/1 -> Demux/1
  Demux/1 -> Terminator11/1
  Demux/3 -> Terminator3/1
  Product/1 -> Fy per wheel/1  "Fy per axe"
  Constant1/1 -> Fx_FR/1
  Constant2/1 -> Fx_FL/1
  Fy per wheel/1 -> Kamm_Circle/3(Fy)
  CK_Factor/1 -> Kamm_Circle/4(CK_Factor)
  Kamm_Circle/3(Fy_R [N] (0,inf)) -> Fy_R [N] (0,inf)/1
  Sum/1 -> Sum2/2, Gravity/1
  Gravity/1 -> Product/2  "Mass [kg]"
  Sum1/1 -> Sum2/1
  Sum2/1 -> Gravity1/1
  Gravity1/1 -> " Mass [kg] (0,inf)"/1
  F_acc/1 -> Demux1/1
  Demux1/3 -> Terminator1/1
  Add/1 -> Handling [-] (-inf,inf)/1
  Demux1/2 -> Add/1
  Constant3/1 -> MATLAB Function1/1(cte)
  Constant4/1 -> MATLAB Function2/1(cte)
  Kamm_Circle/2(Fx_L) -> MATLAB Function1/2(v)
  Demux1/1 -> Integrator/1
  FR_susp/1 -> Sum1/1
  FL_susp/1 -> Sum1/2
  RR_susp/1 -> Sum/1, Kamm_Circle/1(Fz_R)
  RL_susp/1 -> Sum/2, Kamm_Circle/2(Fz_L)
  Kamm_Circle/1(Fx_R) -> MATLAB Function2/2(v)
  Steering_Angle/1 -> Yaw_Rate_Reference/1(Steering_Angle)
  Force Difference with Max. Tire Forces/2(rl_fx) -> "Fx_RL "/1
  Force Difference with Max. Tire Forces/1(rr_fx) -> "Fx_RR "/1
  MATLAB Function2/1(value) -> [Fx_RR]
  MATLAB Function1/1(value) -> [Fx_RL]
  [Fx_RR] -> Force Difference with Max. Tire Forces/2(rr_fx_max)
  [Fx_RL] -> Force Difference with Max. Tire Forces/3(rl_fx_max)
  Yaw_Rate_Reference/1(Yaw_Rate) -> Sum3/1
  Yaw_Rate/1 -> [Yaw_Rate]
  [Yaw_Rate_Ellipse] -> Sum3/2
  Sum3/1 -> Tire Longitudinal Force Difference/1(e)
  Tire Longitudinal Force Difference/1(Fx_diff) -> Force Difference with Max. Tire Forces/1(fx_diff)
  Yaw_Inertia [kg/m^3]/1 -> Tire Longitudinal Force Difference/2(Iz)
  "Rear_Trackwidth [m] "/1 -> Tire Longitudinal Force Difference/4(rt)
  Yaw_error_/dt [s]/1 -> Tire Longitudinal Force Difference/3(dt)
  Constant6/1 -> Flag CarBehavior/1

== system TV_2021/Vehicle Dynamics Control 1/VDC 2018 Complete/Longitudinal Dynamics ==
  F_acc : Inport
  R_acc : Inport  Port=2
  Ellipse_Acc : Inport  Port=3
  FR_susp : Inport  Port=4
  FL_susp : Inport  Port=5
  RR_susp : Inport  Port=6
  RL_susp : Inport  Port=7
  Gas_pedal : Inport  Port=8
  Brake_pedal : Inport  Port=9
  SK_Factor : Inport  Port=10
  Action Port : ActionPort
  Add : Sum  Inputs=++++
  Add1 : Sum  Inputs=-+
  Constant{,1..2,5..6} (5 alike) : Constant  Value=0
  Constant3 : Constant  Value=-1
  Constant4 : Constant  Value=-1
  Demux : Demux  Outputs=3
  Demux1 : Demux  Outputs=3
  Demux2 : Demux  Outputs=3
  Gain : Gain  Gain=1/9.81
  Kamm_Circle : Subsystem
  MATLAB Function : MATLAB Function  TreatAsAtomicUnit=on
  MATLAB Function1 : MATLAB Function  TreatAsAtomicUnit=on
  Terminator{,1..8} (9 alike) : Terminator
  minimum value : MATLAB Function  TreatAsAtomicUnit=on
  Fx_FR : Outport
  Fx_FL : Outport  Port=2
  "Fx_RR " : Outport  Port=3
  "Fx_RL " : Outport  Port=4
  Fy_R : Outport  Port=5
  Mass [kg] (0,inf) : Outport  Port=6
  Handling [-] (-inf,inf) : Outport  Port=7
  Flag CarBehavior : Outport  Port=8
  wires:
  Demux2/1 -> Terminator7/1
  Demux2/3 -> Terminator8/1
  Demux2/2 -> Add1/2
  Ellipse_Acc/1 -> Demux2/1
  Demux/2 -> Terminator/1
  RL_susp/1 -> Add/4, minimum value/2(b)
  RR_susp/1 -> minimum value/1(a), Add/3
  FL_susp/1 -> Add/2
  FR_susp/1 -> Add/1
  Constant6/1 -> Flag CarBehavior/1
  Constant3/1 -> MATLAB Function1/1(cte)
  MATLAB Function1/1(value) -> "Fx_RL "/1
  MATLAB Function/1(value) -> "Fx_RR "/1
  Constant4/1 -> MATLAB Function/1(cte)
  Constant5/1 -> Fy_R/1
  Kamm_Circle/2(Fx_L) -> MATLAB Function1/2(v)
  Kamm_Circle/1(Fx_R) -> MATLAB Function/2(v)
  Demux1/2 -> Add1/1
  Add1/1 -> Handling [-] (-inf,inf)/1
  Demux1/3 -> Terminator1/1
  Demux1/1 -> Terminator2/1
  F_acc/1 -> Demux1/1
  Demux/3 -> Terminator3/1
  Demux/1 -> Terminator6/1
  R_acc/1 -> Demux/1
  Add/1 -> Gain/1
  Gain/1 -> Mass [kg] (0,inf)/1
  minimum value/1(min) -> Kamm_Circle/2(Fz_L), Kamm_Circle/1(Fz_R)
  SK_Factor/1 -> Kamm_Circle/4(SK_Factor)
  Constant/1 -> Kamm_Circle/3(Fy)
  Constant1/1 -> Fx_FR/1
  Constant2/1 -> Fx_FL/1
  Brake_pedal/1 -> Terminator5/1
  Gas_pedal/1 -> Terminator4/1

== system TV_2021/Vehicle Dynamics Control 1/VDC 2018 Complete/Optimization SKF & CKF ==
  RPM_INV1 : Inport
  RPM_INV2 : Inport  Port=2
  Steer_An : Inport  Port=3
  SKF_Initial : Inport  Port=4
  CKF_Initial : Inport  Port=5
  Cte_SKF : Inport  Port=6
  Cte_CKF : Inport  Port=7
  CKF_prev : DataStoreRead  DataStoreName=B
  Constant : Constant  Value=0
  Data Store Memory : DataStoreMemory  ReadBeforeWriteMsg=warning  WriteAfterWriteMsg=warning  WriteAfterReadMsg=warning  ShowAdditionalParam=off
  Data Store Memory1 : DataStoreMemory  DataStoreName=B  ReadBeforeWriteMsg=warning  WriteAfterWriteMsg=warning  WriteAfterReadMsg=warning  ShowAdditionalParam=off
  Data Store Write : DataStoreWrite
  Data Store Write1 : DataStoreWrite  DataStoreName=B
  Derivative : Derivative
  Display : Display
  Display1 : Display
  Display2 : Display
  MATLAB Function : MATLAB Function  TreatAsAtomicUnit=on
  Mux : Mux  Inputs=3
  "SKF_prev " : DataStoreRead
  Saturation : Saturate  UpperLimit=6000  LowerLimit=0
  Scope : Scope
  "Subsystem " : Subsystem
  Switch : Switch  Threshold=900
  SKF_act : Outport
  CKF_act : Outport  Port=2
  wires:
  RPM_INV2/1 -> MATLAB Function/2(RPM_INV2)
  RPM_INV1/1 -> MATLAB Function/1(RPM_INV1), Mux/1
  Constant/1 -> Switch/3
  Switch/1 -> Mux/3
  Saturation/1 -> Mux/2
  Mux/1 -> Scope/1
  MATLAB Function/1(RPM) -> Derivative/1  "w (rad/s)"
  Cte_SKF/1 -> "Subsystem "/7(Cte_SKF)
  CKF_Initial/1 -> "Subsystem "/5("CKF_Initial ")
  Steer_An/1 -> "Subsystem "/1(Steer_An)
  Cte_CKF/1 -> "Subsystem "/8(Cte_CKF)
  "Subsystem "/2(CKF_act) -> Data Store Write1/1, Display2/1, CKF_act/1  "CKF"
  "SKF_prev "/1 -> "Subsystem "/4(SKF_prev)
  Derivative/1 -> "Subsystem "/2(Derivative), Display/1, Saturation/1, Switch/2, Switch/1  "alpha"
  "Subsystem "/1("SKF_act ") -> Data Store Write/1, Display1/1, SKF_act/1  "SKF"
  CKF_prev/1 -> "Subsystem "/6("CKF_prev ")
  SKF_Initial/1 -> "Subsystem "/3(SKF_Initial)

== system TV_2021/Vehicle Dynamics Control 1/VDC 2018 Complete/Sensor_DATA ==
  note: [m/s2]
  note: [rad/s]
  note: [rad/s]
  note: [rad/s]
  note: [0 - Inf]
  note: [0 or 1]
  note: [0-1]
  note: [0-1]
  note: [N]
  note: [N]
  note: [N]
  note: [N]
  note: [deg]
  note: [m/s2]
  note: [m/s2]
  note: [ºC]
  note: [rad/s]
  Steer_Ang : Inport
  "F_Acc " : Inport  Port=2
  R_Acc : Inport  Port=3
  Ellipse_acc : Inport  Port=4
  Yaw Rate : Inport  Port=5
  Gyro_Ellipse : Inport  Port=6
  FR_Susp : Inport  Port=7
  FL_Susp : Inport  Port=8
  RR_Susp : Inport  Port=9
  RL_Susp : Inport  Port=10
  Gas Pedal : Inport  Port=11
  Brake Pedal : Inport  Port=12
  Regenerative Enable : Inport  Port=13
  "Power " : Inport  Port=14
  TemperatureIN : Inport  Port=15
  Temperature Motor : Inport  Port=16
  V_eRR : Inport  Port=17
  "V_eRL " : Inport  Port=18
  Ellipse_vx : Inport  Port=19
  Temp_Celdas : Inport  Port=20
  Limit_Temp_Celdas : Inport  Port=21
  Steer_ang : Outport
  F_acc : Outport  Port=2
  R_acc : Outport  Port=3
  Ellipse_Acc : Outport  Port=4
  YawRate : Outport  Port=5
  GyroEllipse : Outport  Port=6
  FR_susp : Outport  Port=7
  FL_susp : Outport  Port=8
  RR_susp : Outport  Port=9
  RL_susp : Outport  Port=10
  Gas_Pedal : Outport  Port=11
  Brake_Pedal : Outport  Port=12
  Reg_Enable : Outport  Port=13
  Power : Outport  Port=14
  TemperatureIGBT : Outport  Port=15
  TemperatureMotor : Outport  Port=16
  "V_eRR " : Outport  Port=17
  V_eRL : Outport  Port=18
  Ellipse_Vx : Outport  Port=19  VectorParamsAs1DForOutWhenUnconnected=on
  Temp_celdas : Outport  Port=20  VectorParamsAs1DForOutWhenUnconnected=on
  Limit_Temp_celdas : Outport  Port=21  VectorParamsAs1DForOutWhenUnconnected=on
  wires:
  Limit_Temp_Celdas/1 -> Limit_Temp_celdas/1
  Temp_Celdas/1 -> Temp_celdas/1
  Ellipse_vx/1 -> Ellipse_Vx/1
  Ellipse_acc/1 -> Ellipse_Acc/1
  Gyro_Ellipse/1 -> GyroEllipse/1
  Yaw Rate/1 -> YawRate/1
  Temperature Motor/1 -> TemperatureMotor/1
  V_eRR/1 -> "V_eRR "/1
  "V_eRL "/1 -> V_eRL/1
  TemperatureIN/1 -> TemperatureIGBT/1
  "Power "/1 -> Power/1
  Regenerative Enable/1 -> Reg_Enable/1
  Brake Pedal/1 -> Brake_Pedal/1
  Gas Pedal/1 -> Gas_Pedal/1
  "F_Acc "/1 -> F_acc/1
  R_Acc/1 -> R_acc/1
  Steer_Ang/1 -> Steer_ang/1
  FR_Susp/1 -> FR_susp/1
  FL_Susp/1 -> FL_susp/1
  RR_Susp/1 -> RR_susp/1
  RL_Susp/1 -> RL_susp/1

== system TV_2021/Vehicle Dynamics Control 1/VDC 2018 Complete/Wheel_to_engine ==
  "Fx_FR " : Inport
  "Fx_FL " : Inport  Port=2
  "Fx_RR " : Inport  Port=3
  "Fx_RL " : Inport  Port=4
  Re : Inport  Port=5
  RT : Inport  Port=6
  Add : Sum  Inputs=+-
  Constant : Constant  Value=0
  Constant1 : Constant  Value=0
  Fx_to_engineTqRL : Subsystem
  Fx_to_engineTqRR : Subsystem
  MATLAB Function1 : MATLAB Function  TreatAsAtomicUnit=on
  MATLAB Function2 : MATLAB Function  TreatAsAtomicUnit=on
  Tq_diff : Outport  VectorParamsAs1DForOutWhenUnconnected=on
  Tq_FR : Outport  Port=2
  Tq_FL : Outport  Port=3
  Tq_RR : Outport  Port=4
  Tq_RL : Outport  Port=5
  wires:
  Add/1 -> Tq_diff/1
  Constant/1 -> MATLAB Function2/1(cte)
  Constant1/1 -> MATLAB Function1/1(cte)
  MATLAB Function1/1(value) -> Fx_to_engineTqRR/1(Fx)
  MATLAB Function2/1(value) -> Fx_to_engineTqRL/1(Fx)
  "Fx_RR "/1 -> MATLAB Function1/2(v)
  "Fx_RL "/1 -> MATLAB Function2/2(v)
  RT/1 -> Fx_to_engineTqRL/3(RT), Fx_to_engineTqRR/3(RT)
  Re/1 -> Fx_to_engineTqRL/2(Re), Fx_to_engineTqRR/2(Re)
  "Fx_FL "/1 -> Tq_FL/1
  "Fx_FR "/1 -> Tq_FR/1
  Fx_to_engineTqRL/1(Tq) -> Add/2, Tq_RL/1
  Fx_to_engineTqRR/1(Tq) -> Tq_RR/1, Add/1
